simulink model "sm_control_gomx3"  (R2016a)
settings: Solver=VariableStepAuto  StartTime=0.0  StopTime=600  RelTol=1e-3
model workspace: external: MAT-File (data not in the file)
libraries: aausat3_lib x8, vrlib x1
settings Model: Creator=jn  LastModifiedBy=jn
settings DataIOCC: SaveFormat=Array
settings DebuggingCC: SolverPrmCheckMsg=warning  AllowSymbolicDim=off
settings ModelReferenceCC: PropagateSignalLabelsOutOfModel=off
settings ConfigComp: CovModelRefEnable=Off  CovSFcnEnable=off

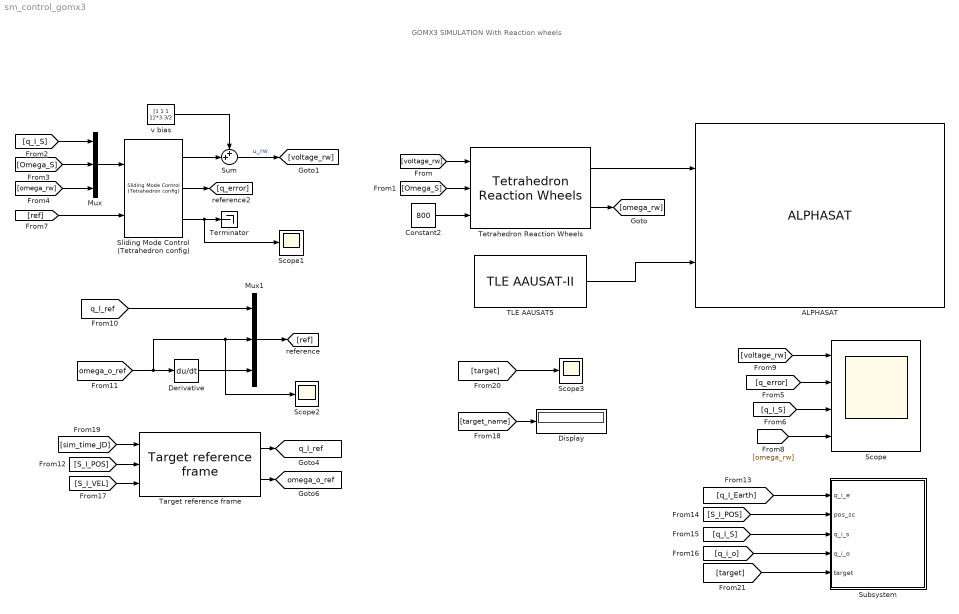
== system sm_control_gomx3 ==
  note: GOMX3 SIMULATION
      | With Reaction wheels
  ALPHASAT : aausat3_lib/ALPHASAT  date='2016-01-05T05:58Z'  q_init_I_S=[0 0 0 1]  w_init_S=[0.02,0.02,0.02]*0  enable_env_disturbance=on  Dim=[0.1 0.1 0.133*3]  sc_mass=3.566  r_com=[-5.238e-8, -0.007e-3, -1.394e-3]  inertia_C=[0.0371 0.0371 0.0059]  q_S_C=[0 0 0 1]  Cd=2  rho=5e-14  solar_m_flux=4.5565e-6  solar_absorb_coeff=1.5
  Constant2 : Constant  Value=800
  Derivative : Derivative
  Display : Display
  Mux : Mux  Inputs=3
  Mux1 : Mux  Inputs=3
  Scope : Scope  NumInputPorts=4
  Scope1 : Scope
  Scope2 : Scope
  Scope3 : Scope
  Sliding Mode Control (Tetrahedron config) : aausat3_lib/ACS/Sliding Mode Control (Tetrahedron config)  K=diag([1 1 1])  delta_0=0.05  e=10e-3  q_s_c=[0 0 0 1]  q_s_tetra=[0 0 1 0]'  max_disturbance=6.0306e-08  enable_coriolis=on  Ts=0.1  Js=[0.0371 0.0371 0.0059]  Jrw=[0.4513 0.4513 0.7]*10^(-6)  Vcc=3.3
  Subsystem : Subsystem  mask{Re=6371e3, scale=1000}
      mask prompts: Re "Earth Radius"; scale "Animation scale"
  Sum : Sum  Inputs=++|
  TLE AAUSAT5 : aausat3_lib/Orbit and Ephemeris/TLE AAUSAT-II  satname='AAUSAT5'  JulianDay=16059.87939624  xndt2o=.00365004  xndd6o=0.61694e-4  bstar=0.10833e-2  xincl=51.6302  xnodeo=228.4109  eo=0.0007308  omegao=258.1510  xmo=101.8678  xno=15.91926461  ts=1
  Target reference frame : aausat3_lib/Orbit and Ephemeris/Target reference frame  min_elevation=5  Ts=10  target_list='target_list.mat'  enabel_target=off
  Terminator : Terminator
  Tetrahedron Reaction Wheels : aausat3_lib/Actuator Emulation/Tetrahedron Reaction Wheels  q_S_Tetra=[0 0 1 0]  I_w=diag([0.4513 0.4513 0.7])*10^(-6)  coriolis_on=on  Kt=1.81e-3  Ke=1.81e-3  Ra=4.44  Vcc=3.3
  v bias : Constant  Value=[1 1 1 1]'*3.3/2
  tag scope: omega_o_ref=global, q_I_ref=global
  wires:
  [voltage_rw] -> Scope/1
  [Omega_S] -> Tetrahedron Reaction Wheels/2
  Tetrahedron Reaction Wheels/1 -> ALPHASAT/1
  Tetrahedron Reaction Wheels/2 -> [omega_rw]
  [q_I_S] -> Mux/1
  [Omega_S] -> Mux/2
  Mux/1 -> Sliding Mode Control (Tetrahedron config)/1
  [q_I_ref] -> Mux1/1
  [omega_rw] -> Mux/3
  Derivative/1 -> Mux1/3
  [q_error] -> Scope/2
  [q_I_S] -> Scope/3
  Sliding Mode Control (Tetrahedron config)/1 -> Sum/2
  v bias/1 -> Sum/1
  Mux1/1 -> [ref]
  [ref] -> Sliding Mode Control (Tetrahedron config)/2
  Sliding Mode Control (Tetrahedron config)/3 -> Scope1/1, Terminator/1
  Constant2/1 -> Tetrahedron Reaction Wheels/3
  [omega_rw] -> Scope/4
  TLE AAUSAT5/1 -> ALPHASAT/2
  [omega_o_ref] -> Derivative/1, Scope2/1, Mux1/2
  Sum/1 -> [voltage_rw]  "u_rw"
  [voltage_rw] -> Tetrahedron Reaction Wheels/1
  Target reference frame/1 -> [q_I_ref]
  [S_I_VEL] -> Target reference frame/3
  [S_I_POS] -> Target reference frame/2
  Target reference frame/2 -> [omega_o_ref]
  [sim_time_JD] -> Target reference frame/1
  [target_name] -> Display/1
  [target] -> Scope3/1
  [q_I_Earth] -> Subsystem/1(q_i_e)
  [S_I_POS] -> Subsystem/2(pos_sc)
  [q_I_S] -> Subsystem/3(q_i_s)
  [q_i_o] -> Subsystem/4(q_i_o)
  [target] -> Subsystem/5(target)
  Sliding Mode Control (Tetrahedron config)/2 -> [q_error]

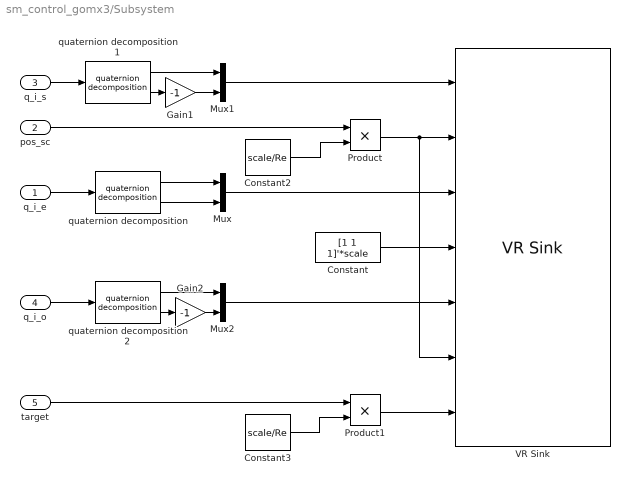
== system sm_control_gomx3/Subsystem ==
  q_i_e : Inport
  pos_sc : Inport  Port=2
  q_i_s : Inport  Port=3
  q_i_o : Inport  Port=4
  target : Inport  Port=5
  Constant : Constant  Value=[1 1 1]'*scale
  Constant2 : Constant  Value=scale/Re
  Constant3 : Constant  Value=scale/Re
  Gain1 : Gain  Gain=-1
  Gain2 : Gain  Gain=-1
  Mux : Mux  Inputs=2
  Mux1 : Mux  Inputs=2
  Mux2 : Mux  Inputs=2
  Product : Product
  Product1 : Product
  VR Sink : vrlib/VR Sink  InstantiateOnLoad=on  SampleTime=0.1  ViewEnable=on  RemoteChange=off  RemoteView=on  FieldsWritten=CubeSat.rotation.4.1.1.double#CubeSat.translation.3.1.1.double#Earth.rotation.4.1.1.double#trans.scale.3.1.1.double#sat_view.rotation.4.1.1.double#sat_view.translation.3.1.1.double#target.translation.3.1.1.double  WorldFileName=lib/utils/animation/sat_orbit.wrl  WorldDescription=The Earth - Low Resolution Model  AutoView=off  VideoDimensions=[]  AllowVariableSize=off
  quaternion decomposition : aausat3_lib/Math Utilities/Quaternion operations/quaternion decomposition
  quaternion decomposition1 : aausat3_lib/Math Utilities/Quaternion operations/quaternion decomposition
  quaternion decomposition2 : aausat3_lib/Math Utilities/Quaternion operations/quaternion decomposition
  wires:
  q_i_e/1 -> quaternion decomposition/1
  quaternion decomposition/2 -> Mux/2
  quaternion decomposition/1 -> Mux/1
  q_i_s/1 -> quaternion decomposition1/1
  quaternion decomposition1/2 -> Gain1/1
  quaternion decomposition1/1 -> Mux1/1
  q_i_o/1 -> quaternion decomposition2/1
  quaternion decomposition2/1 -> Mux2/1
  Gain1/1 -> Mux1/2
  quaternion decomposition2/2 -> Gain2/1
  Gain2/1 -> Mux2/2
  Mux1/1 -> VR Sink/1
  Constant/1 -> VR Sink/4
  pos_sc/1 -> Product/1
  Product/1 -> VR Sink/6, VR Sink/2
  Constant2/1 -> Product/2
  Product1/1 -> VR Sink/7
  Constant3/1 -> Product1/2
  Mux2/1 -> VR Sink/5
  Mux/1 -> VR Sink/3
  target/1 -> Product1/1
